simulink model "model_1"  (R2018a)
settings: Solver=VariableStepAuto  StartTime=0.0  StopTime=10  RelTol=1e-3
values from neighbouring files (symbols this model uses):
  a_0 = 1    [script_1.m]
  a_1 = 1    [script_1.m]
  b = 2    [script_1.m]
  t0 = 1    [script_1.m]
  x0 = 0    [script_1.m]
settings Model: Creator=johnb  LastModifiedBy=johnb

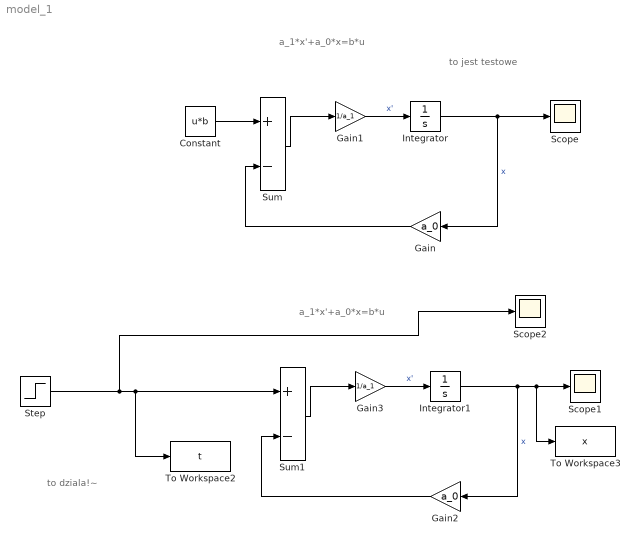
== system model_1 ==
  note: to dziala!~
  note: to jest testowe
  note: a_1*x'+a_0*x=b*u
  note: a_1*x'+a_0*x=b*u
  Constant : Constant  Value=u*b
  Gain : Gain  Gain=a_0
  Gain1 : Gain  Gain=1/a_1
  Gain2 : Gain  Gain=a_0
  Gain3 : Gain  Gain=1/a_1
  Integrator : Integrator  InitialCondition=x0
  Integrator1 : Integrator  InitialCondition=x0
  Scope : Scope
  Scope1 : Scope
  Scope2 : Scope
  Step : Step  Time=t0  Before=x0  After=b*u  SampleTime=0
  Sum : Sum  Inputs=+-
  Sum1 : Sum  Inputs=+-
  To Workspace2 : ToWorkspace  VariableName=t  SaveFormat=Timeseries  SampleTime=-1
  To Workspace3 : ToWorkspace  VariableName=x  SampleTime=-1
  wires:
  Sum/1 -> Gain1/1
  Integrator/1 -> Scope/1, Gain/1  "x"
  Gain1/1 -> Integrator/1  "x'"
  Constant/1 -> Sum/1
  Integrator1/1 -> To Workspace3/1, Scope1/1, Gain2/1  "x"
  Gain3/1 -> Integrator1/1  "x'"
  Sum1/1 -> Gain3/1
  Gain2/1 -> Sum1/2
  Step/1 -> Scope2/1, To Workspace2/1, Sum1/1
  Gain/1 -> Sum/2
